simulink model "Model_Blackbox_system_discrete_PIDs"  (R2024b)
settings: Solver=VariableStepAuto  StartTime=0.0  StopTime=5  RelTol=1e-3
values from neighbouring files (symbols this model uses):
  Beq = 1.0459e-06    [Plant_EstimTrialUpdateLAB17_04_25.m]
  Jeq = 9.8651e-07    [Plant_EstimTrialUpdateLAB17_04_25.m]
  kdrv = 0.6    [Plant_EstimTrialUpdateLAB17_04_25.m]
  ke = 7.68 * 0.001    (= 0.00768)    [Plant_EstimTrialUpdateLAB17_04_25.m]
  Kt = 1.088 * ozin2Nm    (= 0.00768128)    [Plant_EstimTrialUpdateLAB17_04_25.m]
  N = 14    [Plant_EstimTrialUpdateLAB17_04_25.m]
  Req = Ra + Rs    (= 3.1)    [Plant_EstimTrialUpdateLAB17_04_25.m]
  rpm2rads = 2*pi/60    (= 0.10471975512)    [Plant_EstimTrialUpdateLAB17_04_25.m]
  tausf = 0.0061    [Plant_EstimTrialUpdateLAB17_04_25.m]
  Ts = Ts_values(2)    [A_final_measurements.m]    (also in Plant_EstimTrialUpdateLAB17_04_25.m = 0.001)
libraries: simulink x1
settings Model: Creator=Riccardo Grosso  LastModifiedBy=Buton
settings DebuggingCC: AlgebraicLoopMsg=none

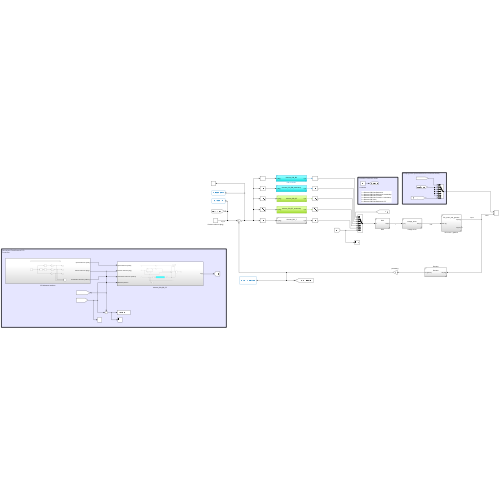
[thumbnail: Simulink's stored preview of the top-level diagram]
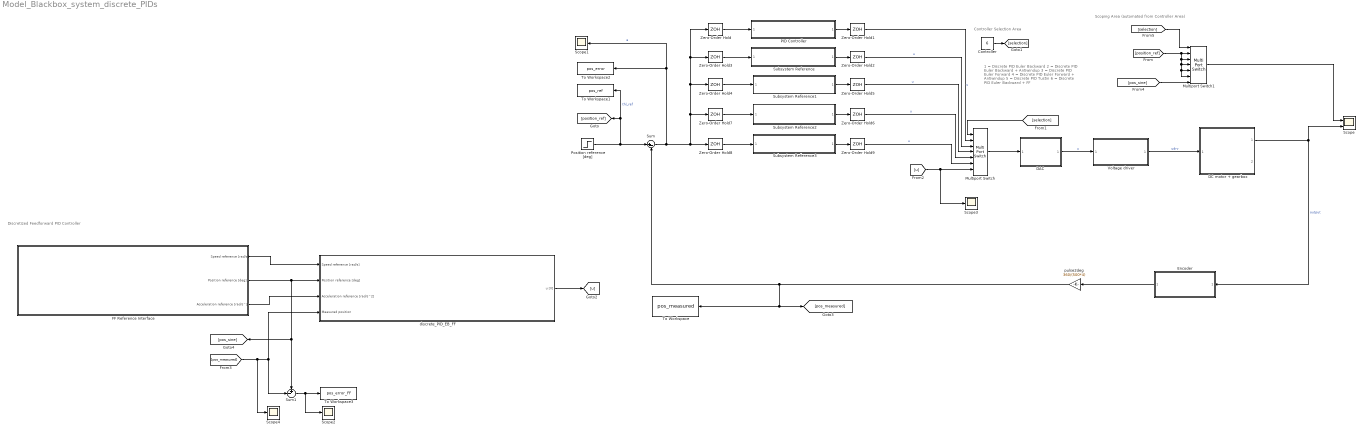
== system Model_Blackbox_system_discrete_PIDs ==
  note: Discretized Feedforward PID
      | Controller
  note: Scoping Area (automated from Controller Area)
  note: 1 = Discrete PID Euler Backward
      | 2 = Discrete PID Euler Backward + Antiwindup
      | 3 = Discrete PID Euler Forward
      | 4 = Discrete PID Euler Forward +  Antiwindup
      | 5 = Discrete PID Tustin
      | 6 = Discrete PID Euler Backward + FF
  note: Controller Selection Area
  Controller : Constant  Value=6
  DAC : Subsystem  ReferencedSubsystem=DAC
  DC motor + gearbox : Subsystem  ReferencedSubsystem=DC_motor_and_gearbox
  Encoder : Subsystem  ReferencedSubsystem=Encoder
  FF Reference Interface : Subsystem
  Multiport Switch : MultiPortSwitch  DataPortOrder=Specify indices  DataPortIndices={1,2,3,4,5,6}  SaturateOnIntegerOverflow=off  InputSameDT=off
  Multiport Switch1 : MultiPortSwitch  DataPortOrder=Specify indices  DataPortIndices={1,2,3,4,5,6}  SaturateOnIntegerOverflow=off  InputSameDT=off
  PID Controller : Subsystem  ReferencedSubsystem=discrete_PID_EB
  Position reference [deg] : Step  After=360  SampleTime=0
  Scope : Scope  NumInputPorts=2
  Scope{1..4} (4 alike) : Scope
  Subsystem Reference : Subsystem  ReferencedSubsystem=discrete_PID_EB_antiwindup
  Subsystem Reference1 : Subsystem  ReferencedSubsystem=discrete_PID_EF
  Subsystem Reference2 : Subsystem  ReferencedSubsystem=discrete_PID_EF_antiwindup
  Subsystem Reference3 : Subsystem  ReferencedSubsystem=discrete_PID_T
  Sum : Sum  Inputs=|+-
  Sum1 : Sum  Inputs=+-|
  To Workspace : ToWorkspace  VariableName=pos_measured  SaveFormat=Timeseries  SampleTime=-1
  To Workspace1 : ToWorkspace  VariableName=pos_ref  SaveFormat=Timeseries  SampleTime=-1
  To Workspace2 : ToWorkspace  VariableName=pos_error  SaveFormat=Timeseries  SampleTime=-1
  To Workspace3 : ToWorkspace  VariableName=pos_error_FF  SaveFormat=Timeseries  SampleTime=-1
  Voltage driver : Subsystem  ReferencedSubsystem=Voltage_driver
  Zero-Order Hold{,1..9} (10 alike) : ZeroOrderHold  SampleTime=Ts
  discrete_PID_EB_FF : Subsystem
  pulse2deg : Gain  Gain=360/(500*4)
  wires:
  Position reference [deg]/1 -> To Workspace1/1, [position_ref], Sum/1  "thl_ref"
  Zero-Order Hold/1 -> PID Controller/1
  PID Controller/1 -> Zero-Order Hold1/1
  DC motor + gearbox/1 -> Scope/2, Encoder/1  "output"
  Subsystem Reference/1 -> Zero-Order Hold2/1
  Zero-Order Hold3/1 -> Subsystem Reference/1
  Sum/1 -> Zero-Order Hold/1, Zero-Order Hold3/1, Zero-Order Hold4/1, Zero-Order Hold7/1, Zero-Order Hold8/1, To Workspace2/1, Scope1/1  "e"
  Zero-Order Hold7/1 -> Subsystem Reference2/1
  Subsystem Reference2/1 -> Zero-Order Hold6/1
  Zero-Order Hold4/1 -> Subsystem Reference1/1
  Subsystem Reference1/1 -> Zero-Order Hold5/1
  Zero-Order Hold8/1 -> Subsystem Reference3/1
  Subsystem Reference3/1 -> Zero-Order Hold9/1
  Multiport Switch/1 -> DAC/1
  Zero-Order Hold1/1 -> Multiport Switch/2  "u"
  Zero-Order Hold2/1 -> Multiport Switch/3  "u"
  Zero-Order Hold5/1 -> Multiport Switch/4  "u"
  Zero-Order Hold6/1 -> Multiport Switch/5  "u"
  Zero-Order Hold9/1 -> Multiport Switch/6  "u"
  [selection] -> Multiport Switch/1
  Controller/1 -> [selection]
  Voltage driver/1 -> DC motor + gearbox/1  "udrv"
  Encoder/1 -> pulse2deg/1
  DAC/1 -> Voltage driver/1  "u"
  pulse2deg/1 -> Sum/2, To Workspace/1, [pos_measured]
  Sum1/1 -> Scope2/1, To Workspace3/1
  FF Reference Interface/1(Speed reference [rad/s]) -> discrete_PID_EB_FF/1(Speed reference [rad/s])
  FF Reference Interface/2(Position reference [deg]1) -> Sum1/1, [pos_sine], discrete_PID_EB_FF/2(Position reference [deg])
  FF Reference Interface/3(Acceleration reference [rad/s^2]) -> discrete_PID_EB_FF/3(Acceleration reference [rad/s^2])
  discrete_PID_EB_FF/1(u [V]) -> [u]
  [u] -> Scope3/1, Multiport Switch/7
  [pos_measured] -> Sum1/2, discrete_PID_EB_FF/4(Measured position), Scope4/1
  [selection] -> Multiport Switch1/1
  Multiport Switch1/1 -> Scope/1
  [pos_sine] -> Multiport Switch1/7
  [position_ref] -> Multiport Switch1/5, Multiport Switch1/6, Multiport Switch1/4, Multiport Switch1/3, Multiport Switch1/2

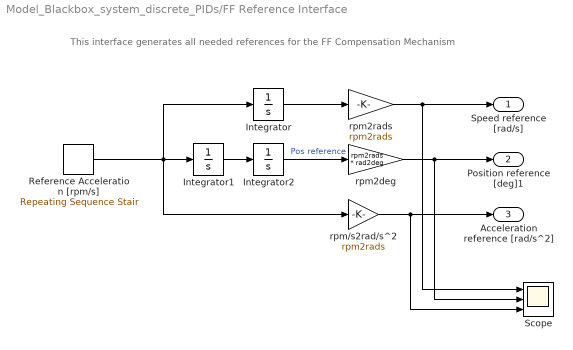
== system Model_Blackbox_system_discrete_PIDs/FF Reference Interface ==
  note: This interface generates all needed references for the FF Compensation Mechanism
  Integrator : Integrator
  Integrator1 : Integrator
  Integrator2 : Integrator
  Reference Acceleration [rpm/s] : simulink/Sources/Repeating Sequence Stair  OutValues=[900 0 -900 -900 0 900].'  tsamp=0.5  OutMin=[]  OutMax=[]  OutDataTypeStr=double  OutputDataTypeScalingMode=double  OutDataType=fixdt(0,8)  ConRadixGroup=Best Precision: Vector-wise  OutScaling=2^-12
  Scope : Scope  NumInputPorts=3
  rpm/s2rad/s^2 : Gain  Gain=rpm2rads
  rpm2deg : Gain  Gain=rpm2rads * rad2deg
  rpm2rads : Gain  Gain=rpm2rads
  Speed reference [rad/s] : Outport
  Position reference [deg]1 : Outport  Port=2
  Acceleration reference [rad/s^2] : Outport  Port=3
  wires:
  Reference Acceleration [rpm/s]/1 -> rpm/s2rad/s^2/1, Integrator1/1, Integrator/1
  Integrator1/1 -> Integrator2/1
  rpm2rads/1 -> Speed reference [rad/s]/1, Scope/1
  Integrator2/1 -> rpm2deg/1  "Pos reference"
  Integrator/1 -> rpm2rads/1
  rpm/s2rad/s^2/1 -> Acceleration reference [rad/s^2]/1, Scope/3
  rpm2deg/1 -> Position reference [deg]1/1, Scope/2

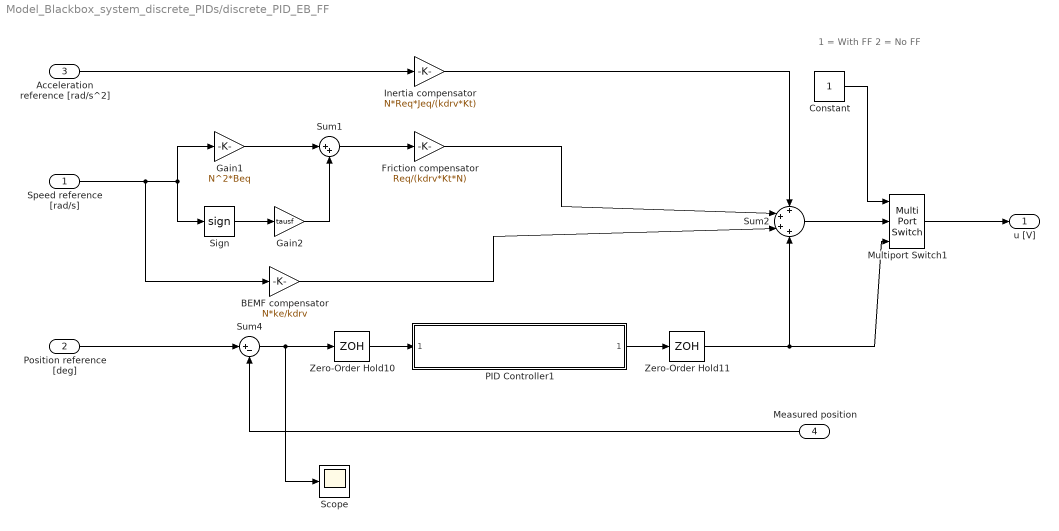
== system Model_Blackbox_system_discrete_PIDs/discrete_PID_EB_FF ==
  note: 1 = With FF
      | 2 = No FF
  Speed reference [rad/s] : Inport
  Position reference [deg] : Inport  Port=2
  Acceleration reference [rad/s^2] : Inport  Port=3
  Measured position : Inport  Port=4
  BEMF compensator : Gain  Gain=N*ke/kdrv
  Constant : Constant
  Friction compensator : Gain  Gain=Req/(kdrv*Kt*N)
  Gain1 : Gain  Gain=N^2*Beq
  Gain2 : Gain  Gain=tausf
  Inertia compensator : Gain  Gain=N*Req*Jeq/(kdrv*Kt)
  Multiport Switch1 : MultiPortSwitch  Inputs=2  SaturateOnIntegerOverflow=off  InputSameDT=off
  PID Controller1 : Subsystem  ReferencedSubsystem=discrete_PID_EB
  Scope : Scope
  Sign : Signum
  Sum1 : Sum  Inputs=|++
  Sum2 : Sum  Inputs=++++
  Sum4 : Sum  Inputs=|+-
  Zero-Order Hold10 : ZeroOrderHold  SampleTime=Ts
  Zero-Order Hold11 : ZeroOrderHold  SampleTime=Ts
  u [V] : Outport
  wires:
  Measured position/1 -> Sum4/2
  Inertia compensator/1 -> Sum2/1
  Sign/1 -> Gain2/1
  Multiport Switch1/1 -> u [V]/1
  Speed reference [rad/s]/1 -> BEMF compensator/1, Sign/1, Gain1/1
  BEMF compensator/1 -> Sum2/3
  PID Controller1/1 -> Zero-Order Hold11/1
  Acceleration reference [rad/s^2]/1 -> Inertia compensator/1
  Gain2/1 -> Sum1/2
  Gain1/1 -> Sum1/1
  Sum1/1 -> Friction compensator/1
  Zero-Order Hold11/1 -> Multiport Switch1/3, Sum2/4
  Constant/1 -> Multiport Switch1/1
  Zero-Order Hold10/1 -> PID Controller1/1
  Friction compensator/1 -> Sum2/2
  Position reference [deg]/1 -> Sum4/1
  Sum4/1 -> Scope/1, Zero-Order Hold10/1
  Sum2/1 -> Multiport Switch1/2
